simulink model "Control_test"  (R2014b)
settings: Solver=FixedStepDiscrete  StartTime=0.0  StopTime=Inf  FixedStep=0.001  RelTol=1e-3
PostLoadFcn:
  | , if any(exist('dsrtsu_mdlpostloadfcn', 'file') == [2, 3, 6]), try dsrtsu_mdlpostloadfcn('Execute', bdroot); catch fprintf('Error in PostLoadFcn (dsrtsu_mdlpostloadfcn) for model "%s":\n %s\n', bdroot, lasterr); end, end,
undefined symbols (not defined in the file or in its folder): dtLocal, slcm
libraries: rtican x163, simulink x14
(part 8 of 34)

== system Control_test/OutputProcessing/SPAS5 ==
  T_Spas_Stat : Inport
  T_Spas_TM_CTRL_Mode : Inport  Port=2
  T_Spas_TM_Cmd : Inport  Port=3
  T_Spas_AliveCnt : Inport  Port=4
  L_SPAS5 : rtican/RTICAN Transmit (TX)   Reserved1=[]  Reserved2=[]  Reserved3=[]  Reserved4=[]  SfcnMessage=[]  Msg_Struct=[]  BoardTypeNo=[]  BoardNo=[]  ChannelNo=[]  Parameters=[]  DialogFcn=[]  UnitName=[]  Revision=[]  UnitValues=[]  DSProperties=struct('RTI',struct('Version',uint32(5),'BlockType',struct('isSLSource',uint8(1),'isSLSink',uint8(1),'isHWSource',uint8(0),'isHWSink',uint8(0),'isSetup',uint8(0),'isInline',uint8(1),'isNonInline',uint8(0),'isInterrupt',uint8(0),'isChannelwise',uint8(0)),'IOBoardType','RTICAN','UnitType','MESSAGE','Identifier','TX','DialogType','MSVC','BlockSet','RTICAN','SlaveProcessor','CAN'))  RTIBlockInterface=struct('InputPortsWidth',int32([1 1 1 1]),'InputPortsActive',[1 1 1 1],'InputPortsName',{{'T_Spas_Stat','T_Spas_TM_CTRL_Mode','T_Spas_TM_Cmd','T_Spas_AliveCnt'}},'InputPortsDataType',{{'SS_DOUBLE','SS_DOUBLE','SS_DOUBLE','SS_DOUBLE'}},'OutputPortsWidth',int32(0),'OutputPortsActive',0,'OutputPortsName',{{''}},'DialogFcn','rtican_message_interface_gui','BlockDisplay',{{'','center'}},'IconTransparency','on','InitLevel',3,'BlockName',struct('Token',{{'L_SPAS5'}}),'SampleTime',{{0.1}},'TriggerPort',{{'none'}},'EnablePort',{{'none'}})  RTIBlockParameters=struct('BoardTypeNo',{{1,'OFF',[]}},'BoardNo',{{1,'ON',[1 16]}},'ChannelNo',{{1,'ON',[1 2]}},'Parameters',{{struct('DataFileSupport',struct('DataFileSelectedMaster',1,'DataFileSelectedLocal',1,'DataFileName',['c:\users\mpc\dropbox\hyundai car setup\01_dbc_files\hmc_can_for_ucb_v2.dbc|c:\users\mpc\dropbox\hyundai car setup\mobileye spec new\mobileye_mando_camera_ucb_v2.dbc|'],'DataFileDate',{{{['26-Nov-2014 10:54:28']},{['18-Sep-2013 10:55:24']}}},'SelectedFile','c:\users\mpc_car\documents\github\mpc-car\dbcfiles\hmc_can_for_ucb_v2.dbc'),'Options',struct('StatusSelected',0,'TimeSelected',0,'DeltaTimeSelected',0,'DelayTimeSelected',0,'DelayTimeTXCommandSelected',0,'EncodeSetUnusedBitsToOne',0,'EnableMsgLoopback',0,'TriggerPort',struct('Selected',0,'TriggerType',0),'EnablePortSelected',0,'SignalOnPortnameSelected',1,'UserCoding',struct('Selected',0,'InterfaceFile','UserEncodingFile','FcnName','UserEncodeFcn','InportSelected',0,'InportWidth',1,'OutportSelected',0,'OutportWidth',1),'TerminationMsg',struct('Selected',0,'Byte0_7','0'),'InitialMsg',struct('Selected',0,'Byte0_7','0')),'Message',struct('MsgOnBlocknameSelected',1,'MsgName','L_SPAS5','MsgIdFormat',0,'MsgId',1584,'MsgLength',8,'NumSignals',4,'SampleTime',0.1,'StartTime',struct('Selected',0,'Value',0),'AutoRepeatTime',struct('Selected',0,'Value',0.1),'Timeout',struct('Selected',0,'Value',0.1),'DelayTime',struct('Selected',0,'Value',0.1),'Signal',struct('SgnName',{'T_Spas_Stat','T_Spas_TM_CTRL_Mode','T_Spas_TM_Cmd','T_Spas_AliveCnt'},'SgnStartBit',{0,8,16,24},'SgnLength',{4,4,4,8},'SgnType',{0,0,0,0},'ModeValue',{-1,-1,-1,-1},'DataType',{1,1,1,0},'ByteLayout',{0,0,0,0},'Factor',{1,1,1,1},'Offset',{0,0,0,0},'SgnComment',{{''},{''},{''},{''}},'SgnUnit',{'','','',''},'Min',{0,0,0,0},'Max',{0,0,0,0},'SLDataType',{'SS_DOUBLE','SS_DOUBLE','SS_DOUBLE','SS_DOUBLE'}),'MsgIdNumFormat',1,'MsgComment',{{''}}),'Version',1.2,'general',struct('isFromLib',0)),'OFF',[]}},'GroupId',{{struct('Group',{{'RTICAN'}},'No',1,'Behavior',{{'NAMECHANGE'}},'BlockType',{{'SINK'}},'NameChangeFlag',0),'OFF',[]}},'SFcnRTICANMessage',{{struct('MsgType','TX','SFcnPortType','Scalar','MsgName','L_SPAS5','MsgIdFormat','STD','MsgId',1584,'MsgLength',8,'NumSignals',4,'SampleTime',0.1,'StartTime',struct('Selected','no','Value',0),'AutoRepeatTime',struct('Selected','no','Value',0.1),'Timeout',struct('Selected','no','Value',0.1),'Signal',struct('SgnName',{'T_Spas_Stat','T_Spas_TM_CTRL_Mode','T_Spas_TM_Cmd','T_Spas_AliveCnt'},'SgnStartBit',{0,8,16,24},'SgnLength',{4,4,4,8},'SgnType',{'standard','standard','standard','standard'},'ModeValue',{-1,-1,-1,-1},'DataType',{['signed int'],['signed int'],['signed int'],['unsigned int']},'ByteLayout',{['little endian'],['little endian'],['little endian'],['little endian']},'Factor',{1,1,1,1},'Offset',{0,0,0,0},'SLDataType',{'SS_DOUBLE','SS_DOUBLE','SS_DOUBLE','SS_DOUBLE'}),'StatusSelected','no','TimeSelected','no','DeltaTimeSelected','no','DelayTimeSelected','no','DelayTimeTXCommandSelected','no','EncodeSetUnusedBitsToOne','no','EnableMsgLoopback','no','TriggerPort',struct('Selected','no','TriggerType',0),'EnablePortSelected','no','UserCoding',struct('Selected','no','InterfaceFile','UserEncodingFile','FcnName','UserEncodeFcn','InportSelected','no','InportWidth',1,'OutportSelected','no','OutportWidth',1),'TerminationMsg',struct('Selected','no','Byte0','0x00','Byte1','0x00','Byte2','0x00','Byte3','0x00','Byte4','0x00','Byte5','0x00','Byte6','0x00','Byte7','0x00'),'InitialMsg',struct('Selected','no','Byte0','0x00','Byte1','0x00','Byte2','0x00','Byte3','0x00','Byte4','0x00','Byte5','0x00','Byte6','0x00','Byte7','0x00'),'BoardType','DS1','BoardNo',1,'ControllerNo',1),'OFF',[]}},'TLCFileName',{{'rtican_tx_message','OFF',[]}})  RTISFcnParameters=struct('SFcnRTICANMessage','struct','TLCFileName','char')  RTIBlockParaDefault=struct('BoardTypeNo',4302,'BoardNo',1,'ChannelNo',1,'Parameters',struct('DataFileSupport',struct('DataFileSelectedMaster',0,'DataFileSelectedLocal',0,'DataFileName','','DataFileDate','','SelectedFile',['<no file selected>']),'Options',struct('StatusSelected',1,'TimeSelected',1,'DeltaTimeSelected',1,'DelayTimeSelected',1,'DelayTimeTXCommandSelected',0,'EncodeSetUnusedBitsToOne',0,'EnableMsgLoopback',0,'TriggerPort',struct('Selected',0,'TriggerType','rising'),'EnablePortSelected',0,'SignalOnPortnameSelected',1,'UserCoding',struct('Selected',0,'InterfaceFile','UserEncodingFile','FcnName','UserEncodeFcn','InportSelected',0,'InportWidth',1,'OutportSelected',0,'OutportWidth',1),'TerminationMsg',struct('Selected',0,'Byte0_7','0'),'InitialMsg',struct('Selected',0,'Byte0_7','0')),'Message',struct('MsgOnBlocknameSelected',0,'MsgName',['TX Message'],'MsgIdFormat',0,'MsgId',100,'MsgLength',8,'NumSignals',1,'SampleTime',-1,'StartTime',struct('Selected',0,'Value',0),'AutoRepeatTime',struct('Selected',0,'Value',0.1),'Timeout',struct('Selected',0,'Value',0.1),'DelayTime',struct('Selected',0,'Value',0.1),'Signal',struct('SgnName',['TX signal'],'SgnStartBit',0,'SgnLength',8,'SgnType',0,'ModeValue',-1,'DataType',0,'SLDataType','SS_DOUBLE','ByteLayout',0,'Factor',1,'Offset',0,'Min',0,'Max',255,'SgnComment',{{}},'SgnUnit',''),'MsgIdNumFormat',0,'MsgComment',{{''}}),'Version',1.2,'general',struct('isFromLib',1)),'GroupId',struct('Group',{{'RTICAN'}},'No',1,'Behavior',{{'NAMECHANGE'}},'BlockType',{{'SINK'}},'NameChangeFlag',0),'SFcnRTICANMessage',struct('MsgType','TX','MsgName',['TX Message'],'MsgIdFormat','STD','MsgId',100,'MsgLength',2,'NumSignals',1,'SampleTime',-1,'StartTime',struct('Selected','no','Value',0),'AutoRepeatTime',struct('Selected','no','Value',0.1),'Timeout',struct('Selected','no','Value',0.1),'DelayTime',struct('Selected','no','Value',0.1),'Signal',struct('SgnName',['TX signal'],'SgnStartBit',0,'SgnLength',8,'SgnType','standard','ModeValue',-1,'DataType',['unsigned int'],'ByteLayout',['little endian'],'SLDataType','SS_DOUBLE','Factor',1,'Offset',0),'StatusSelected','yes','TimeSelected','yes','DeltaTimeSelected','yes','DelayTimeSelected','yes','EnablePortSelected','no','EnableMsgLoopback','no','DelayTimeTXCommandSelected','no','EncodeSetUnusedBitsToOne','no','UserCoding',struct('Selected','no','InterfaceFile','UserDecodingFile','FcnName','UserDecodeFcn','InportSelected','no','InportWidth',1,'OutportSelected','no','OutportWidth',1),'TerminationMsg',struct('Selected','no','Byte0','0x00','Byte1','0x00','Byte2','0x00','Byte3','0x00','Byte4','0x00','Byte5','0x00','Byte6','0x00','Byte7','0x00'),'InitialMsg',struct('Selected','no','Byte0','0x00','Byte1','0x00','Byte2','0x00','Byte3','0x00','Byte4','0x00','Byte5','0x00','Byte6','0x00','Byte7','0x00'),'TriggerPort',struct('Selected','no','TriggerType','rising'),'BoardType','DS4302','BoardNo',1,'ControllerNo',1,'SFcnPortType','Scalar'),'TLCFileName','rtican_tx_message')
      settings: AttributesFormatString=Group Id: RTICAN1\n
  Rate Transition{1..4} (4 alike) : RateTransition  OutPortSampleTime=0.1
  wires:
  T_Spas_Stat/1 -> Rate Transition4/1
  T_Spas_TM_CTRL_Mode/1 -> Rate Transition3/1
  T_Spas_TM_Cmd/1 -> Rate Transition1/1
  Rate Transition1/1 -> L_SPAS5/3
  Rate Transition3/1 -> L_SPAS5/2
  Rate Transition4/1 -> L_SPAS5/1
  Rate Transition2/1 -> L_SPAS5/4
  T_Spas_AliveCnt/1 -> Rate Transition2/1

== system Control_test/OutputProcessing/TM_AliveCnt ==
  Trigger : TriggerPort  PortDimensions=1
  Add : Sum
  Constant : Constant
  Constant1 : Constant  Value=0
  Switch1 : Switch  Criteria=u2 > Threshold  Threshold=255
  Unit Delay : UnitDelay  SampleTime=-1
  T_Spas_AliveCnt : Outport
  wires:
  Constant/1 -> Add/1
  Constant1/1 -> Switch1/1
  Add/1 -> Switch1/2, Switch1/3
  Switch1/1 -> Unit Delay/1, T_Spas_AliveCnt/1
  Unit Delay/1 -> Add/2

== system Control_test/OutputProcessing/VehicleCanProcessing ==
  In1 : Inport
  delta_f [rad] : Inport  Port=2
  DriverOverride_flag : Inport  Port=3
  torque [Nm] : Inport  Port=4
  " " : Gain
  " 1" : Gain
  Active Flag : Constant  Value=0
  Add : Sum
  Add1 : Sum
  Bus Selector : BusSelector  OutputSignals=Vehicle Data.EMS1.ipEmsVehSpd[kph],Vehicle Data.SAS1Data.ipStrAng[deg]
  GearRatio : Gain  Gain=14.5
  LKAS2 : Subsystem
  Req Steering Angle [deg] : Constant  Value=0
  Saturation : Saturate  UpperLimit=360  LowerLimit=-360
  Switch1 : Switch  Threshold=0.5
  default1 : Constant  Value=0
  rad2deg : Gain  Gain=(180/pi)
  steerOffDeg : Constant  Value=0
  tag scope: SteerActiveFlag=global
  wires:
  In1/1 -> Bus Selector/1
  Bus Selector/1 -> LKAS2/3(Vs)  "<ipEmsVehSpd[kph]>"
  Bus Selector/2 -> LKAS2/4(SteeringAngle)  "<ipStrAng[deg]>"
  Req Steering Angle [deg]/1 -> " 1"/1
  Add/1 -> LKAS2/1(Req Steering Angle[deg])
  " "/1 -> LKAS2/2(Active_Flag)  "in_enable"
  " 1"/1 -> Add/2  "Req_Steering_Angle_deg"
  Add1/1 -> Add/1
  delta_f [rad]/1 -> rad2deg/1
  rad2deg/1 -> GearRatio/1
  Switch1/1 -> " "/1
  default1/1 -> Switch1/1
  DriverOverride_flag/1 -> Switch1/2
  Active Flag/1 -> Switch1/3, [SteerActiveFlag]
  GearRatio/1 -> Saturation/1
  Saturation/1 -> Add1/1  "commanded_steering"
  steerOffDeg/1 -> Add1/2
  torque [Nm]/1 -> LKAS2/5(Req Steering Tq [Nm])

== system Control_test/RTI Data/RTI Data Store ==
  RTI Data Store : Subsystem  mask(RTI_DATA_STORE){}
      mask help:
      | RTI Data Store Block. This block is used by RTI to store internal model dependent data. Deleting this block will result in data loss.
      |
      | NEVER DELETE, COPY, OR MODIFY THIS BLOCK!
      mask Help:
      | RTI Data Store Block. This block is used by RTI to store internal model dependent data. Deleting this block will result in data loss.
      | 
      | NEVER DELETE, COPY, OR MODIFY THIS BLOCK!
      mask Display: text(0.5, 0.5, ' ', 'HorizontalAlignment', 'center');

== system Control_test/SensorFusion/Map-based Localization ==
  In1 : Inport
  Add : Sum
  Bus Selector1 : BusSelector  OutputSignals=IMU_data.signal2.PosLon,IMU_data.signal2.PosLat,IMU_data.signal1.AngleHeading,Vehicle Data.WhlSpdData.ipVehSpdWhl[m/s]
  INS Reference Change : MATLAB Function
      settings: RTWSystemCode=Inline
  Mux1 : Mux  Inputs=3
  Mux4 : Mux  Inputs=2
  OffsetX : Constant  Value=0
  OffsetY : Constant  Value=0
  gain1 : Gain
  gain2 : Gain
  OutMap : Outport
  wires:
  Add/1 -> Mux1/1
  OffsetY/1 -> gain2/1
  OffsetX/1 -> gain1/1
  Mux4/1 -> Add/1
  gain1/1 -> Mux4/1  "MapOffsetX"
  gain2/1 -> Mux4/2  "MapOffsetY"
  In1/1 -> Bus Selector1/1
  INS Reference Change/1(GPS_Local_Pos) -> Add/2
  INS Reference Change/2(INS_Heading) -> Mux1/2
  Bus Selector1/4 -> Mux1/3  "<ipVehSpdWhl[m/s]>"
  Bus Selector1/1 -> INS Reference Change/1(PosLon)  "<PosLon>"
  Bus Selector1/2 -> INS Reference Change/2(PosLat)  "<PosLat>"
  Bus Selector1/3 -> INS Reference Change/3(AngleHeading)  "<AngleHeading>"
  Mux1/1 -> OutMap/1

== system Control_test/InputProcessing/CameraCanProcessing/ME_Lane_Additional_Data_1 ==
  Bus Creator : BusCreator  Inputs=14
  ME_Lane_Additional_Data_1 : rtican/RTICAN Receive (RX)   Reserved1=[]  Reserved2=[]  Reserved3=[]  Reserved4=[]  SfcnMessage=[]  Msg_Struct=[]  BoardTypeNo=[]  BoardNo=[]  ChannelNo=[]  Parameters=[]  DialogFcn=[]  UnitName=[]  Revision=[]  UnitValues=[]  DSProperties=struct('RTI',struct('Version',uint32(5),'BlockType',struct('isSLSource',uint8(1),'isSLSink',uint8(1),'isHWSource',uint8(0),'isHWSink',uint8(0),'isSetup',uint8(0),'isInline',uint8(1),'isNonInline',uint8(0),'isInterrupt',uint8(0),'isChannelwise',uint8(0)),'IOBoardType','RTICAN','UnitType','MESSAGE','Identifier','RX','DialogType','MSVC','BlockSet','RTICAN','SlaveProcessor','CAN'))  RTIBlockInterface=struct('OutputPortsWidth',int32([1 1 1 1 1 1 1 1 1 1 1 1 1 1]),'OutputPortsActive',[1 1 1 1 1 1 1 1 1 1 1 1 1 1],'OutputPortsName',{{'Rh_Neightbor_Avail','Lh_Neightbor_Avail','Rh_Neightbor_Type','Lh_Neightbor_Type','Alive_Counter_MELaneAddData','Rh_Guardrail','Lh_Guardrail','RightLanePrediction','LeftLanePrediction','HighwayExit','RightLaneColorInfo','LeftLaneColorInfo','Lh_ViewRange_StartPoint','Rh_ViewRange_StartPoint'}},'OutputPortsDataType',{{'SS_DOUBLE','SS_DOUBLE','SS_DOUBLE','SS_DOUBLE','SS_DOUBLE','SS_DOUBLE','SS_DOUBLE','SS_DOUBLE','SS_DOUBLE','SS_DOUBLE','SS_DOUBLE','SS_DOUBLE','SS_DOUBLE','SS_DOUBLE'}},'OutputPortsLabel',{{'Rh_Neightbor_Avail','Lh_Neightbor_Avail','Rh_Neightbor_Type','Lh_Neightbor_Type','Alive_Counter_MELaneAddData','Rh_Guardrail','Lh_Guardrail','RightLanePrediction','LeftLanePrediction','HighwayExit','RightLaneColorInfo','LeftLaneColorInfo','Lh_ViewRange_StartPoint','Rh_ViewRange_StartPoint'}},'OutputPortsLabelMode','ON','InputPortsWidth',int32(0),'InputPortsActive',0,'DialogFcn','rtican_message_interface_gui','BlockDisplay',{{'','center'}},'IconTransparency','on','ParameterTunableNames',{{}},'InitLevel',3,'BlockName',struct('Token',{{'ME_Lane_Additional_Data_1'}}),'SampleTime',{{0.01}},'TriggerPort',{{'none'}},'EnablePort',{{'none'}})  RTIBlockParameters=struct('BoardTypeNo',{{1,'OFF',[]}},'BoardNo',{{1,'ON',[1 16]}},'ChannelNo',{{2,'ON',[1 2]}},'Parameters',{{struct('DataFileSupport',struct('DataFileSelectedMaster',1,'DataFileSelectedLocal',1,'DataFileName',['c:\users\mpc\desktop\hyundai car setup\rt2000_can_mod.dbc|c:\users\mpc\desktop\hyundai car setup\mobileye spec new\mobileye_mando_camera_ucb_v2.dbc|'],'DataFileDate',['18-Sep-2013 17:55:24'],'SelectedFile','..\..\dbcfiles\mobileye_mando_camera_ucb_v2.dbc','InterfaceFcn','rtican_dbc_file_parser'),'Options',struct('StatusSelected',0,'TimeSelected',0,'DeltaTimeSelected',0,'BytePortSelected',0,'MessageLengthSelected',0,'TriggerPort',struct('Selected',0,'TriggerType',0),'UserCoding',struct('Selected',0,'InterfaceFile','UserDecodingFile','FcnName','UserDecodeFcn','InportSelected',0,'InportWidth',1,'OutportSelected',0,'OutportWidth',1),'EnablePortSelected',0,'SignalOnPortnameSelected',1,'UseRXService',0),'Message',struct('MsgOnBlocknameSelected',1,'MsgName','ME_Lane_Additional_Data_1','MsgIdFormat',0,'MsgId',1901,'MsgLength',8,'NumSignals',14,'SampleTime',0.01,'Signal',struct('SgnName',{'Rh_Neightbor_Avail','Lh_Neightbor_Avail','Rh_Neightbor_Type','Lh_Neightbor_Type','Alive_Counter_MELaneAddData','Rh_Guardrail','Lh_Guardrail','RightLanePrediction','LeftLanePrediction','HighwayExit','RightLaneColorInfo','LeftLaneColorInfo','Lh_ViewRange_StartPoint','Rh_ViewRange_StartPoint'},'SgnStartBit',{0,4,8,12,16,18,19,24,25,26,28,30,32,48},'SgnLength',{4,4,4,4,2,1,1,1,1,1,2,2,16,16},'ByteLayout',{0,0,0,0,0,0,0,0,0,0,0,0,0,0},'Factor',{1,1,1,1,1,1,1,1,1,1,1,1,0.01,0.01},'Offset',{0,0,0,0,0,0,0,0,0,0,0,0,0,0},'SgnComment',{'','','','','','','','','','','','','',''},'SgnUnit',{'','','','','','','','','','','','','',''},'Min',{0,0,0,0,0,0,0,0,0,0,0,0,0,0},'Max',{0,0,0,0,0,0,0,0,0,0,0,0,0,0},'SgnType',{0,0,0,0,0,0,0,0,0,0,0,0,0,0},'SLDataType',{'SS_DOUBLE','SS_DOUBLE','SS_DOUBLE','SS_DOUBLE','SS_DOUBLE','SS_DOUBLE','SS_DOUBLE','SS_DOUBLE','SS_DOUBLE','SS_DOUBLE','SS_DOUBLE','SS_DOUBLE','SS_DOUBLE','SS_DOUBLE'},'DataType',{0,0,0,0,0,0,0,0,0,0,0,0,0,0},'ModeValue',{-1,-1,-1,-1,-1,-1,-1,-1,-1,-1,-1,-1,-1,-1}),'MsgIdNumFormat',0,'MsgComment',{{''}}),'Version',1.2,'general',struct('isFromLib',0)),'OFF',[]}},'GroupId',{{struct('Group',{{'RTICAN'}},'No',2,'Behavior',{{'NAMECHANGE'}},'BlockType',{{'SINK'}},'NameChangeFlag',0),'OFF',[]}},'SFcnRTICANMessage',{{struct('MsgType','RX','SFcnPortType','Scalar','MsgName','ME_Lane_Additional_Data_1','MsgIdFormat','STD','MsgId',1901,'MsgLength',8,'NumSignals',14,'SampleTime',0.01,'Signal',struct('SgnName',{'Rh_Neightbor_Avail','Lh_Neightbor_Avail','Rh_Neightbor_Type','Lh_Neightbor_Type','Alive_Counter_MELaneAddData','Rh_Guardrail','Lh_Guardrail','RightLanePrediction','LeftLanePrediction','HighwayExit','RightLaneColorInfo','LeftLaneColorInfo','Lh_ViewRange_StartPoint','Rh_ViewRange_StartPoint'},'SgnStartBit',{0,4,8,12,16,18,19,24,25,26,28,30,32,48},'SgnLength',{4,4,4,4,2,1,1,1,1,1,2,2,16,16},'ByteLayout',{['little endian'],['little endian'],['little endian'],['little endian'],['little endian'],['little endian'],['little endian'],['little endian'],['little endian'],['little endian'],['little endian'],['little endian'],['little endian'],['little endian']},'Factor',{1,1,1,1,1,1,1,1,1,1,1,1,0.01,0.01},'Offset',{0,0,0,0,0,0,0,0,0,0,0,0,0,0},'SgnType',{'standard','standard','standard','standard','standard','standard','standard','standard','standard','standard','standard','standard','standard','standard'},'SLDataType',{'SS_DOUBLE','SS_DOUBLE','SS_DOUBLE','SS_DOUBLE','SS_DOUBLE','SS_DOUBLE','SS_DOUBLE','SS_DOUBLE','SS_DOUBLE','SS_DOUBLE','SS_DOUBLE','SS_DOUBLE','SS_DOUBLE','SS_DOUBLE'},'DataType',{['unsigned int'],['unsigned int'],['unsigned int'],['unsigned int'],['unsigned int'],['unsigned int'],['unsigned int'],['unsigned int'],['unsigned int'],['unsigned int'],['unsigned int'],['unsigned int'],['unsigned int'],['unsigned int']},'ModeValue',{-1,-1,-1,-1,-1,-1,-1,-1,-1,-1,-1,-1,-1,-1}),'StatusSelected','no','TimeSelected','no','DeltaTimeSelected','no','BytePortSelected','no','MessageLengthSelected','no','TriggerPort',struct('Selected','no','TriggerType',0),'UserCoding',struct('Selected','no','InterfaceFile','UserDecodingFile','FcnName','UserDecodeFcn','InportSelected','no','InportWidth',1,'OutportSelected','no','OutportWidth',1),'EnablePortSelected','no','UseRXService','no','BoardType','DS1','BoardNo',1,'ControllerNo',2),'OFF',[]}},'TLCFileName',{{'rtican_rx_message','OFF',[]}})  RTISFcnParameters=struct('SFcnRTICANMessage','struct','TLCFileName','char')  RTIBlockParaDefault=struct('BoardTypeNo',4302,'BoardNo',1,'ChannelNo',1,'Parameters',struct('DataFileSupport',struct('DataFileSelectedMaster',0,'DataFileSelectedLocal',0,'DataFileName','','DataFileDate','','SelectedFile',['<no file selected>']),'Options',struct('StatusSelected',1,'TimeSelected',1,'DeltaTimeSelected',1,'BytePortSelected',0,'MessageLengthSelected',0,'TriggerPort',struct('Selected',0,'TriggerType','rising'),'UserCoding',struct('Selected',0,'InterfaceFile','UserDecodingFile','FcnName','UserDecodeFcn','InportSelected',0,'InportWidth',1,'OutportSelected',0,'OutportWidth',1),'EnablePortSelected',0,'SignalOnPortnameSelected',1,'UseRXService',0),'Message',struct('MsgOnBlocknameSelected',0,'MsgName',['RX Message'],'MsgIdFormat',0,'MsgId',100,'MsgLength',8,'NumSignals',1,'SampleTime',-1,'Signal',struct('SgnName',['RX signal'],'SgnStartBit',0,'SgnLength',8,'SgnType',0,'ModeValue',-1,'DataType',0,'SLDataType','SS_DOUBLE','ByteLayout',0,'Factor',1,'Offset',0,'Min',0,'Max',255,'SgnComment',{{}},'SgnUnit',''),'MsgIdNumFormat',0,'MsgComment',{{''}}),'Version',1.2,'general',struct('isFromLib',1)),'GroupId',struct('Group',{{'RTICAN'}},'No',1,'Behavior',{{'NAMECHANGE'}},'BlockType',{{'SINK'}},'NameChangeFlag',0),'SFcnRTICANMessage',struct('MsgType','RX','MsgName',['RX Message'],'MsgIdFormat','STD','MsgId',100,'MsgLength',8,'NumSignals',1,'SampleTime',-1,'Signal',struct('SgnName',['RX signal'],'SgnStartBit',0,'SgnLength',8,'SgnType','standard','ModeValue',-1,'DataType',['unsigned int'],'ByteLayout',['little endian'],'SLDataType','SS_DOUBLE','Factor',1,'Offset',0),'StatusSelected','yes','TimeSelected','yes','DeltaTimeSelected','yes','BytePortSelected','no','MessageLengthSelected','no','EnablePortSelected','no','UserCoding',struct('Selected','no','InterfaceFile','UserDecodingFile','FcnName','UserDecodeFcn','InportSelected','no','InportWidth',1,'OutportSelected','no','OutportWidth',1),'TriggerPort',struct('Selected','no','TriggerType','rising'),'UseRXService','no','BoardType','DS4302','BoardNo',1,'ControllerNo',1,'SFcnPortType','Scalar'),'TLCFileName','rtican_rx_message')
      settings: AttributesFormatString=Group Id: RTICAN2\n
  ME_Lane_Additional_Data_1_CAN : Outport
  wires:
  Bus Creator/1 -> ME_Lane_Additional_Data_1_CAN/1
  ME_Lane_Additional_Data_1/1 -> Bus Creator/1  "Rh_Neightbor_Avail"
  ME_Lane_Additional_Data_1/2 -> Bus Creator/2  "Lh_Neightbor_Avail"
  ME_Lane_Additional_Data_1/3 -> Bus Creator/3  "Rh_Neightbor_Type"
  ME_Lane_Additional_Data_1/4 -> Bus Creator/4  "Lh_Neightbor_Type"
  ME_Lane_Additional_Data_1/5 -> Bus Creator/5  "Alive_Counter_MELaneAddData"
  ME_Lane_Additional_Data_1/6 -> Bus Creator/6  "Rh_Guardrail"
  ME_Lane_Additional_Data_1/7 -> Bus Creator/7  "Lh_Guardrail"
  ME_Lane_Additional_Data_1/8 -> Bus Creator/8  "RightLanePrediction"
  ME_Lane_Additional_Data_1/9 -> Bus Creator/9  "LeftLanePrediction"
  ME_Lane_Additional_Data_1/10 -> Bus Creator/10  "HighwayExit"
  ME_Lane_Additional_Data_1/11 -> Bus Creator/11  "RightLaneColorInfo"
  ME_Lane_Additional_Data_1/12 -> Bus Creator/12  "LeftLaneColorInfo"
  ME_Lane_Additional_Data_1/13 -> Bus Creator/13  "Lh_ViewRange_StartPoint"
  ME_Lane_Additional_Data_1/14 -> Bus Creator/14  "Rh_ViewRange_StartPoint"

== system Control_test/InputProcessing/CameraCanProcessing/ME_Lane_Additional_Data_2 ==
  Bus Creator : BusCreator  Inputs=5
  ME_Lane_Additional_Data_2 : rtican/RTICAN Receive (RX)   Reserved1=[]  Reserved2=[]  Reserved3=[]  Reserved4=[]  SfcnMessage=[]  Msg_Struct=[]  BoardTypeNo=[]  BoardNo=[]  ChannelNo=[]  Parameters=[]  DialogFcn=[]  UnitName=[]  Revision=[]  UnitValues=[]  DSProperties=struct('RTI',struct('Version',uint32(5),'BlockType',struct('isSLSource',uint8(1),'isSLSink',uint8(1),'isHWSource',uint8(0),'isHWSink',uint8(0),'isSetup',uint8(0),'isInline',uint8(1),'isNonInline',uint8(0),'isInterrupt',uint8(0),'isChannelwise',uint8(0)),'IOBoardType','RTICAN','UnitType','MESSAGE','Identifier','RX','DialogType','MSVC','BlockSet','RTICAN','SlaveProcessor','CAN'))  RTIBlockInterface=struct('OutputPortsWidth',int32([1 1 1 1 1]),'OutputPortsActive',[1 1 1 1 1],'OutputPortsName',{{'Alive_Counter_MELaneAddData','Lh_Neighbor_Pos','Lh_Neighbor_Model_B','Lh_Neighbor_Model_A','Lh_Neighbor_Model_dA'}},'OutputPortsDataType',{{'SS_DOUBLE','SS_DOUBLE','SS_DOUBLE','SS_DOUBLE','SS_DOUBLE'}},'OutputPortsLabel',{{'Alive_Counter_MELaneAddData','Lh_Neighbor_Pos','Lh_Neighbor_Model_B','Lh_Neighbor_Model_A','Lh_Neighbor_Model_dA'}},'OutputPortsLabelMode','ON','InputPortsWidth',int32(0),'InputPortsActive',0,'DialogFcn','rtican_message_interface_gui','BlockDisplay',{{'','center'}},'IconTransparency','on','ParameterTunableNames',{{}},'InitLevel',3,'BlockName',struct('Token',{{'ME_Lane_Additional_Data_2'}}),'SampleTime',{{0.01}},'TriggerPort',{{'none'}},'EnablePort',{{'none'}})  RTIBlockParameters=struct('BoardTypeNo',{{1,'OFF',[]}},'BoardNo',{{1,'ON',[1 16]}},'ChannelNo',{{2,'ON',[1 2]}},'Parameters',{{struct('DataFileSupport',struct('DataFileSelectedMaster',1,'DataFileSelectedLocal',1,'DataFileName',['c:\users\mpc\desktop\hyundai car setup\rt2000_can_mod.dbc|c:\users\mpc\desktop\hyundai car setup\mobileye spec new\mobileye_mando_camera_ucb_v2.dbc|'],'DataFileDate',['18-Sep-2013 17:55:24'],'SelectedFile','..\..\dbcfiles\mobileye_mando_camera_ucb_v2.dbc','InterfaceFcn','rtican_dbc_file_parser'),'Options',struct('StatusSelected',0,'TimeSelected',0,'DeltaTimeSelected',0,'BytePortSelected',0,'MessageLengthSelected',0,'TriggerPort',struct('Selected',0,'TriggerType',0),'UserCoding',struct('Selected',0,'InterfaceFile','UserDecodingFile','FcnName','UserDecodeFcn','InportSelected',0,'InportWidth',1,'OutportSelected',0,'OutportWidth',1),'EnablePortSelected',0,'SignalOnPortnameSelected',1,'UseRXService',0),'Message',struct('MsgOnBlocknameSelected',1,'MsgName','ME_Lane_Additional_Data_2','MsgIdFormat',0,'MsgId',1902,'MsgLength',8,'NumSignals',5,'SampleTime',0.01,'Signal',struct('SgnName',{'Alive_Counter_MELaneAddData','Lh_Neighbor_Pos','Lh_Neighbor_Model_B','Lh_Neighbor_Model_A','Lh_Neighbor_Model_dA'},'SgnStartBit',{0,8,16,32,48},'SgnLength',{2,8,16,16,16},'ByteLayout',{0,0,0,0,0},'Factor',{1,0.05,1,1,1},'Offset',{0,0,0,0,0},'SgnComment',{'','','','',''},'SgnUnit',{'','','','',''},'Min',{0,0,0,0,0},'Max',{0,0,0,0,0},'SgnType',{0,0,0,0,0},'SLDataType',{'SS_DOUBLE','SS_DOUBLE','SS_DOUBLE','SS_DOUBLE','SS_DOUBLE'},'DataType',{0,0,1,1,1},'ModeValue',{-1,-1,-1,-1,-1}),'MsgIdNumFormat',0,'MsgComment',{{''}}),'Version',1.2,'general',struct('isFromLib',0)),'OFF',[]}},'GroupId',{{struct('Group',{{'RTICAN'}},'No',2,'Behavior',{{'NAMECHANGE'}},'BlockType',{{'SINK'}},'NameChangeFlag',0),'OFF',[]}},'SFcnRTICANMessage',{{struct('MsgType','RX','SFcnPortType','Scalar','MsgName','ME_Lane_Additional_Data_2','MsgIdFormat','STD','MsgId',1902,'MsgLength',8,'NumSignals',5,'SampleTime',0.01,'Signal',struct('SgnName',{'Alive_Counter_MELaneAddData','Lh_Neighbor_Pos','Lh_Neighbor_Model_B','Lh_Neighbor_Model_A','Lh_Neighbor_Model_dA'},'SgnStartBit',{0,8,16,32,48},'SgnLength',{2,8,16,16,16},'ByteLayout',{['little endian'],['little endian'],['little endian'],['little endian'],['little endian']},'Factor',{1,0.05,1,1,1},'Offset',{0,0,0,0,0},'SgnType',{'standard','standard','standard','standard','standard'},'SLDataType',{'SS_DOUBLE','SS_DOUBLE','SS_DOUBLE','SS_DOUBLE','SS_DOUBLE'},'DataType',{['unsigned int'],['unsigned int'],['signed int'],['signed int'],['signed int']},'ModeValue',{-1,-1,-1,-1,-1}),'StatusSelected','no','TimeSelected','no','DeltaTimeSelected','no','BytePortSelected','no','MessageLengthSelected','no','TriggerPort',struct('Selected','no','TriggerType',0),'UserCoding',struct('Selected','no','InterfaceFile','UserDecodingFile','FcnName','UserDecodeFcn','InportSelected','no','InportWidth',1,'OutportSelected','no','OutportWidth',1),'EnablePortSelected','no','UseRXService','no','BoardType','DS1','BoardNo',1,'ControllerNo',2),'OFF',[]}},'TLCFileName',{{'rtican_rx_message','OFF',[]}})  RTISFcnParameters=struct('SFcnRTICANMessage','struct','TLCFileName','char')  RTIBlockParaDefault=struct('BoardTypeNo',4302,'BoardNo',1,'ChannelNo',1,'Parameters',struct('DataFileSupport',struct('DataFileSelectedMaster',0,'DataFileSelectedLocal',0,'DataFileName','','DataFileDate','','SelectedFile',['<no file selected>']),'Options',struct('StatusSelected',1,'TimeSelected',1,'DeltaTimeSelected',1,'BytePortSelected',0,'MessageLengthSelected',0,'TriggerPort',struct('Selected',0,'TriggerType','rising'),'UserCoding',struct('Selected',0,'InterfaceFile','UserDecodingFile','FcnName','UserDecodeFcn','InportSelected',0,'InportWidth',1,'OutportSelected',0,'OutportWidth',1),'EnablePortSelected',0,'SignalOnPortnameSelected',1,'UseRXService',0),'Message',struct('MsgOnBlocknameSelected',0,'MsgName',['RX Message'],'MsgIdFormat',0,'MsgId',100,'MsgLength',8,'NumSignals',1,'SampleTime',-1,'Signal',struct('SgnName',['RX signal'],'SgnStartBit',0,'SgnLength',8,'SgnType',0,'ModeValue',-1,'DataType',0,'SLDataType','SS_DOUBLE','ByteLayout',0,'Factor',1,'Offset',0,'Min',0,'Max',255,'SgnComment',{{}},'SgnUnit',''),'MsgIdNumFormat',0,'MsgComment',{{''}}),'Version',1.2,'general',struct('isFromLib',1)),'GroupId',struct('Group',{{'RTICAN'}},'No',1,'Behavior',{{'NAMECHANGE'}},'BlockType',{{'SINK'}},'NameChangeFlag',0),'SFcnRTICANMessage',struct('MsgType','RX','MsgName',['RX Message'],'MsgIdFormat','STD','MsgId',100,'MsgLength',8,'NumSignals',1,'SampleTime',-1,'Signal',struct('SgnName',['RX signal'],'SgnStartBit',0,'SgnLength',8,'SgnType','standard','ModeValue',-1,'DataType',['unsigned int'],'ByteLayout',['little endian'],'SLDataType','SS_DOUBLE','Factor',1,'Offset',0),'StatusSelected','yes','TimeSelected','yes','DeltaTimeSelected','yes','BytePortSelected','no','MessageLengthSelected','no','EnablePortSelected','no','UserCoding',struct('Selected','no','InterfaceFile','UserDecodingFile','FcnName','UserDecodeFcn','InportSelected','no','InportWidth',1,'OutportSelected','no','OutportWidth',1),'TriggerPort',struct('Selected','no','TriggerType','rising'),'UseRXService','no','BoardType','DS4302','BoardNo',1,'ControllerNo',1,'SFcnPortType','Scalar'),'TLCFileName','rtican_rx_message')
      settings: AttributesFormatString=Group Id: RTICAN2\n
  ME_Lane_Additional_Data_2_CAN : Outport
  wires:
  Bus Creator/1 -> ME_Lane_Additional_Data_2_CAN/1
  ME_Lane_Additional_Data_2/1 -> Bus Creator/1  "Alive_Counter_MELaneAddData"
  ME_Lane_Additional_Data_2/2 -> Bus Creator/2  "Lh_Neighbor_Pos"
  ME_Lane_Additional_Data_2/3 -> Bus Creator/3  "Lh_Neighbor_Model_B"
  ME_Lane_Additional_Data_2/4 -> Bus Creator/4  "Lh_Neighbor_Model_A"
  ME_Lane_Additional_Data_2/5 -> Bus Creator/5  "Lh_Neighbor_Model_dA"

== system Control_test/InputProcessing/CameraCanProcessing/ME_Lane_Additional_Data_3 ==
  Bus Creator : BusCreator  Inputs=5
  ME_Lane_Additional_Data_3 : rtican/RTICAN Receive (RX)   Reserved1=[]  Reserved2=[]  Reserved3=[]  Reserved4=[]  SfcnMessage=[]  Msg_Struct=[]  BoardTypeNo=[]  BoardNo=[]  ChannelNo=[]  Parameters=[]  DialogFcn=[]  UnitName=[]  Revision=[]  UnitValues=[]  DSProperties=struct('RTI',struct('Version',uint32(5),'BlockType',struct('isSLSource',uint8(1),'isSLSink',uint8(1),'isHWSource',uint8(0),'isHWSink',uint8(0),'isSetup',uint8(0),'isInline',uint8(1),'isNonInline',uint8(0),'isInterrupt',uint8(0),'isChannelwise',uint8(0)),'IOBoardType','RTICAN','UnitType','MESSAGE','Identifier','RX','DialogType','MSVC','BlockSet','RTICAN','SlaveProcessor','CAN'))  RTIBlockInterface=struct('OutputPortsWidth',int32([1 1 1 1 1]),'OutputPortsActive',[1 1 1 1 1],'OutputPortsName',{{'Alive_Counter_MELaneAddData','Rh_Neighbor_Pos','Rh_Neighbor_Model_B','Rh_Neighbor_Model_A','Rh_Neighbor_Model_dA'}},'OutputPortsDataType',{{'SS_DOUBLE','SS_DOUBLE','SS_DOUBLE','SS_DOUBLE','SS_DOUBLE'}},'OutputPortsLabel',{{'Alive_Counter_MELaneAddData','Rh_Neighbor_Pos','Rh_Neighbor_Model_B','Rh_Neighbor_Model_A','Rh_Neighbor_Model_dA'}},'OutputPortsLabelMode','ON','InputPortsWidth',int32(0),'InputPortsActive',0,'DialogFcn','rtican_message_interface_gui','BlockDisplay',{{'','center'}},'IconTransparency','on','ParameterTunableNames',{{}},'InitLevel',3,'BlockName',struct('Token',{{'ME_Lane_Additional_Data_3'}}),'SampleTime',{{0.01}},'TriggerPort',{{'none'}},'EnablePort',{{'none'}})  RTIBlockParameters=struct('BoardTypeNo',{{1,'OFF',[]}},'BoardNo',{{1,'ON',[1 16]}},'ChannelNo',{{2,'ON',[1 2]}},'Parameters',{{struct('DataFileSupport',struct('DataFileSelectedMaster',1,'DataFileSelectedLocal',0,'DataFileName',['c:\users\mpc\dropbox\hyundai car setup\dbc files\rt2002_can.dbc|c:\users\mpc\dropbox\cpg_test_2014\t4_rfs_demo\hyundai car setup\mobileye spec new\mobileye_mando_camera_ucb_v2.dbc|'],'DataFileDate',{{{['13-Nov-2012 16:29:35']},{['18-Sep-2013 10:55:24']}}},'SelectedFile',['<no file selected>'],'InterfaceFcn','rtican_dbc_file_parser'),'Options',struct('StatusSelected',0,'TimeSelected',0,'DeltaTimeSelected',0,'BytePortSelected',0,'MessageLengthSelected',0,'TriggerPort',struct('Selected',0,'TriggerType',0),'UserCoding',struct('Selected',0,'InterfaceFile','UserDecodingFile','FcnName','UserDecodeFcn','InportSelected',0,'InportWidth',1,'OutportSelected',0,'OutportWidth',1),'EnablePortSelected',0,'SignalOnPortnameSelected',1,'UseRXService',0),'Message',struct('MsgOnBlocknameSelected',1,'MsgName','ME_Lane_Additional_Data_3','MsgIdFormat',0,'MsgId',1903,'MsgLength',8,'NumSignals',5,'SampleTime',0.01,'Signal',struct('SgnName',{'Alive_Counter_MELaneAddData','Rh_Neighbor_Pos','Rh_Neighbor_Model_B','Rh_Neighbor_Model_A','Rh_Neighbor_Model_dA'},'SgnStartBit',{0,8,16,32,48},'SgnLength',{2,8,16,16,16},'SgnType',{0,0,0,0,0},'ModeValue',{-1,-1,-1,-1,-1},'DataType',{0,0,0,0,0},'ByteLayout',{0,0,0,0,0},'Factor',{1,0.05,0.0009765,0.01,3.725e-09},'Offset',{0,0,31.999,0,0.00012206},'SgnComment',{{''},{''},{''},{''},{''}},'SgnUnit',{'','','','',''},'Min',{0,0,0,0,0},'Max',{0,0,0,0,0},'SLDataType',{'SS_DOUBLE','SS_DOUBLE','SS_DOUBLE','SS_DOUBLE','SS_DOUBLE'}),'MsgIdNumFormat',0,'MsgComment',{{''}}),'Version',1.2,'general',struct('isFromLib',0)),'OFF',[]}},'GroupId',{{struct('Group',{{'RTICAN'}},'No',2,'Behavior',{{'NAMECHANGE'}},'BlockType',{{'SINK'}},'NameChangeFlag',0),'OFF',[]}},'SFcnRTICANMessage',{{struct('MsgType','RX','SFcnPortType','Scalar','MsgName','ME_Lane_Additional_Data_3','MsgIdFormat','STD','MsgId',1903,'MsgLength',8,'NumSignals',5,'SampleTime',0.01,'Signal',struct('SgnName',{'Alive_Counter_MELaneAddData','Rh_Neighbor_Pos','Rh_Neighbor_Model_B','Rh_Neighbor_Model_A','Rh_Neighbor_Model_dA'},'SgnStartBit',{0,8,16,32,48},'SgnLength',{2,8,16,16,16},'SgnType',{'standard','standard','standard','standard','standard'},'ModeValue',{-1,-1,-1,-1,-1},'DataType',{['unsigned int'],['unsigned int'],['unsigned int'],['unsigned int'],['unsigned int']},'ByteLayout',{['little endian'],['little endian'],['little endian'],['little endian'],['little endian']},'Factor',{1,0.05,0.0009765,0.01,3.725e-09},'Offset',{0,0,31.999,0,0.00012206},'SLDataType',{'SS_DOUBLE','SS_DOUBLE','SS_DOUBLE','SS_DOUBLE','SS_DOUBLE'}),'StatusSelected','no','TimeSelected','no','DeltaTimeSelected','no','BytePortSelected','no','MessageLengthSelected','no','TriggerPort',struct('Selected','no','TriggerType',0),'UserCoding',struct('Selected','no','InterfaceFile','UserDecodingFile','FcnName','UserDecodeFcn','InportSelected','no','InportWidth',1,'OutportSelected','no','OutportWidth',1),'EnablePortSelected','no','UseRXService','no','BoardType','DS1','BoardNo',1,'ControllerNo',2),'OFF',[]}},'TLCFileName',{{'rtican_rx_message','OFF',[]}})  RTISFcnParameters=struct('SFcnRTICANMessage','struct','TLCFileName','char')  RTIBlockParaDefault=struct('BoardTypeNo',4302,'BoardNo',1,'ChannelNo',1,'Parameters',struct('DataFileSupport',struct('DataFileSelectedMaster',0,'DataFileSelectedLocal',0,'DataFileName','','DataFileDate','','SelectedFile',['<no file selected>']),'Options',struct('StatusSelected',1,'TimeSelected',1,'DeltaTimeSelected',1,'BytePortSelected',0,'MessageLengthSelected',0,'TriggerPort',struct('Selected',0,'TriggerType','rising'),'UserCoding',struct('Selected',0,'InterfaceFile','UserDecodingFile','FcnName','UserDecodeFcn','InportSelected',0,'InportWidth',1,'OutportSelected',0,'OutportWidth',1),'EnablePortSelected',0,'SignalOnPortnameSelected',1,'UseRXService',0),'Message',struct('MsgOnBlocknameSelected',0,'MsgName',['RX Message'],'MsgIdFormat',0,'MsgId',100,'MsgLength',8,'NumSignals',1,'SampleTime',-1,'Signal',struct('SgnName',['RX signal'],'SgnStartBit',0,'SgnLength',8,'SgnType',0,'ModeValue',-1,'DataType',0,'SLDataType','SS_DOUBLE','ByteLayout',0,'Factor',1,'Offset',0,'Min',0,'Max',255,'SgnComment',{{}},'SgnUnit',''),'MsgIdNumFormat',0,'MsgComment',{{''}}),'Version',1.2,'general',struct('isFromLib',1)),'GroupId',struct('Group',{{'RTICAN'}},'No',1,'Behavior',{{'NAMECHANGE'}},'BlockType',{{'SINK'}},'NameChangeFlag',0),'SFcnRTICANMessage',struct('MsgType','RX','MsgName',['RX Message'],'MsgIdFormat','STD','MsgId',100,'MsgLength',8,'NumSignals',1,'SampleTime',-1,'Signal',struct('SgnName',['RX signal'],'SgnStartBit',0,'SgnLength',8,'SgnType','standard','ModeValue',-1,'DataType',['unsigned int'],'ByteLayout',['little endian'],'SLDataType','SS_DOUBLE','Factor',1,'Offset',0),'StatusSelected','yes','TimeSelected','yes','DeltaTimeSelected','yes','BytePortSelected','no','MessageLengthSelected','no','EnablePortSelected','no','UserCoding',struct('Selected','no','InterfaceFile','UserDecodingFile','FcnName','UserDecodeFcn','InportSelected','no','InportWidth',1,'OutportSelected','no','OutportWidth',1),'TriggerPort',struct('Selected','no','TriggerType','rising'),'UseRXService','no','BoardType','DS4302','BoardNo',1,'ControllerNo',1,'SFcnPortType','Scalar'),'TLCFileName','rtican_rx_message')
      settings: AttributesFormatString=Group Id: RTICAN2\n
  ME_Lane_Additional_Data_3_CAN : Outport
  wires:
  Bus Creator/1 -> ME_Lane_Additional_Data_3_CAN/1
  ME_Lane_Additional_Data_3/1 -> Bus Creator/1  "Alive_Counter_MELaneAddData"
  ME_Lane_Additional_Data_3/2 -> Bus Creator/2  "Rh_Neighbor_Pos"
  ME_Lane_Additional_Data_3/3 -> Bus Creator/3  "Rh_Neighbor_Model_B"
  ME_Lane_Additional_Data_3/4 -> Bus Creator/4  "Rh_Neighbor_Model_A"
  ME_Lane_Additional_Data_3/5 -> Bus Creator/5  "Rh_Neighbor_Model_dA"

== system Control_test/InputProcessing/CameraCanProcessing/ME_Left_Lane_A ==
  Bus Creator : BusCreator  Inputs=7
  ME_Left_Lane_A : rtican/RTICAN Receive (RX)   Reserved1=[]  Reserved2=[]  Reserved3=[]  Reserved4=[]  SfcnMessage=[]  Msg_Struct=[]  BoardTypeNo=[]  BoardNo=[]  ChannelNo=[]  Parameters=[]  DialogFcn=[]  UnitName=[]  Revision=[]  UnitValues=[]  DSProperties=struct('RTI',struct('Version',uint32(5),'BlockType',struct('isSLSource',uint8(1),'isSLSink',uint8(1),'isHWSource',uint8(0),'isHWSink',uint8(0),'isSetup',uint8(0),'isInline',uint8(1),'isNonInline',uint8(0),'isInterrupt',uint8(0),'isChannelwise',uint8(0)),'IOBoardType','RTICAN','UnitType','MESSAGE','Identifier','RX','DialogType','MSVC','BlockSet','RTICAN','SlaveProcessor','CAN'))  RTIBlockInterface=struct('OutputPortsWidth',int32([1 1 1 1 1 1 1]),'OutputPortsActive',[1 1 1 1 1 1 1],'OutputPortsName',{{'LaneMarkType_Lh_ME','LaneMarkQuality_Lh_ME','LDW_Warning_Lh_ME','LDW_Availability_Lh_ME','LaneMarkPosition_Lh_ME','LaneMarkModelA_Lh_ME','LaneMarkWidth_Lh_ME'}},'OutputPortsDataType',{{'SS_DOUBLE','SS_DOUBLE','SS_DOUBLE','SS_DOUBLE','SS_DOUBLE','SS_DOUBLE','SS_DOUBLE'}},'OutputPortsLabel',{{'LaneMarkType_Lh_ME','LaneMarkQuality_Lh_ME','LDW_Warning_Lh_ME','LDW_Availability_Lh_ME','LaneMarkPosition_Lh_ME','LaneMarkModelA_Lh_ME','LaneMarkWidth_Lh_ME'}},'OutputPortsLabelMode','ON','InputPortsWidth',int32(0),'InputPortsActive',0,'DialogFcn','rtican_message_interface_gui','BlockDisplay',{{'','center'}},'IconTransparency','on','ParameterTunableNames',{{}},'InitLevel',3,'BlockName',struct('Token',{{'ME_Left_Lane_A'}}),'SampleTime',{{0.01}},'TriggerPort',{{'none'}},'EnablePort',{{'none'}})  RTIBlockParameters=struct('BoardTypeNo',{{1,'OFF',[]}},'BoardNo',{{1,'ON',[1 16]}},'ChannelNo',{{2,'ON',[1 2]}},'Parameters',{{struct('DataFileSupport',struct('DataFileSelectedMaster',1,'DataFileSelectedLocal',0,'DataFileName',['c:\users\mpc\dropbox\cpg_test_2014\t4_rfs_demo\hyundai car setup\rt2000_can_mod.dbc|c:\users\mpc\dropbox\cpg_test_2014\t4_rfs_demo\hyundai car setup\mobileye spec new\mobileye_mando_camera_ucb_v2.dbc|'],'DataFileDate',{{{['13-Nov-2012 16:29:35']},{['18-Sep-2013 10:55:24']}}},'SelectedFile',['<no file selected>'],'InterfaceFcn','rtican_dbc_file_parser'),'Options',struct('StatusSelected',0,'TimeSelected',0,'DeltaTimeSelected',0,'BytePortSelected',0,'MessageLengthSelected',0,'TriggerPort',struct('Selected',0,'TriggerType',0),'UserCoding',struct('Selected',0,'InterfaceFile','UserDecodingFile','FcnName','UserDecodeFcn','InportSelected',0,'InportWidth',1,'OutportSelected',0,'OutportWidth',1),'EnablePortSelected',0,'SignalOnPortnameSelected',1,'UseRXService',0),'Message',struct('MsgOnBlocknameSelected',1,'MsgName','ME_Left_Lane_A','MsgIdFormat',0,'MsgId',1894,'MsgLength',8,'NumSignals',7,'SampleTime',0.01,'Signal',struct('SgnName',{'LaneMarkType_Lh_ME','LaneMarkQuality_Lh_ME','LDW_Warning_Lh_ME','LDW_Availability_Lh_ME','LaneMarkPosition_Lh_ME','LaneMarkModelA_Lh_ME','LaneMarkWidth_Lh_ME'},'SgnStartBit',{0,4,6,7,8,24,56},'SgnLength',{4,2,1,1,16,32,8},'SgnType',{0,0,0,0,0,0,0},'ModeValue',{-1,-1,-1,-1,-1,-1,-1},'DataType',{0,0,0,0,1,0,0},'ByteLayout',{0,0,0,0,0,0,0},'Factor',{1,1,1,1,0.00390625,2.3283064e-10,0.005},'Offset',{0,0,0,0,0,-0.5,0},'SgnComment',{{''},{''},{''},{''},{''},{''},{''}},'SgnUnit',{'','','','','','1/Meters',''},'Min',{0,0,0,0,0,0,0},'Max',{0,0,0,0,0,0,0},'SLDataType',{'SS_DOUBLE','SS_DOUBLE','SS_DOUBLE','SS_DOUBLE','SS_DOUBLE','SS_DOUBLE','SS_DOUBLE'}),'MsgIdNumFormat',1,'MsgComment',{{''}}),'Version',1.2,'general',struct('isFromLib',0)),'OFF',[]}},'GroupId',{{struct('Group',{{'RTICAN'}},'No',2,'Behavior',{{'NAMECHANGE'}},'BlockType',{{'SINK'}},'NameChangeFlag',0),'OFF',[]}},'SFcnRTICANMessage',{{struct('MsgType','RX','SFcnPortType','Scalar','MsgName','ME_Left_Lane_A','MsgIdFormat','STD','MsgId',1894,'MsgLength',8,'NumSignals',7,'SampleTime',0.01,'Signal',struct('SgnName',{'LaneMarkType_Lh_ME','LaneMarkQuality_Lh_ME','LDW_Warning_Lh_ME','LDW_Availability_Lh_ME','LaneMarkPosition_Lh_ME','LaneMarkModelA_Lh_ME','LaneMarkWidth_Lh_ME'},'SgnStartBit',{0,4,6,7,8,24,56},'SgnLength',{4,2,1,1,16,32,8},'SgnType',{'standard','standard','standard','standard','standard','standard','standard'},'ModeValue',{-1,-1,-1,-1,-1,-1,-1},'DataType',{['unsigned int'],['unsigned int'],['unsigned int'],['unsigned int'],['signed int'],['unsigned int'],['unsigned int']},'ByteLayout',{['little endian'],['little endian'],['little endian'],['little endian'],['little endian'],['little endian'],['little endian']},'Factor',{1,1,1,1,0.00390625,2.3283064e-10,0.005},'Offset',{0,0,0,0,0,-0.5,0},'SLDataType',{'SS_DOUBLE','SS_DOUBLE','SS_DOUBLE','SS_DOUBLE','SS_DOUBLE','SS_DOUBLE','SS_DOUBLE'}),'StatusSelected','no','TimeSelected','no','DeltaTimeSelected','no','BytePortSelected','no','MessageLengthSelected','no','TriggerPort',struct('Selected','no','TriggerType',0),'UserCoding',struct('Selected','no','InterfaceFile','UserDecodingFile','FcnName','UserDecodeFcn','InportSelected','no','InportWidth',1,'OutportSelected','no','OutportWidth',1),'EnablePortSelected','no','UseRXService','no','BoardType','DS1','BoardNo',1,'ControllerNo',2),'OFF',[]}},'TLCFileName',{{'rtican_rx_message','OFF',[]}})  RTISFcnParameters=struct('SFcnRTICANMessage','struct','TLCFileName','char')  RTIBlockParaDefault=struct('BoardTypeNo',4302,'BoardNo',1,'ChannelNo',1,'Parameters',struct('DataFileSupport',struct('DataFileSelectedMaster',0,'DataFileSelectedLocal',0,'DataFileName','','DataFileDate','','SelectedFile',['<no file selected>']),'Options',struct('StatusSelected',1,'TimeSelected',1,'DeltaTimeSelected',1,'BytePortSelected',0,'MessageLengthSelected',0,'TriggerPort',struct('Selected',0,'TriggerType','rising'),'UserCoding',struct('Selected',0,'InterfaceFile','UserDecodingFile','FcnName','UserDecodeFcn','InportSelected',0,'InportWidth',1,'OutportSelected',0,'OutportWidth',1),'EnablePortSelected',0,'SignalOnPortnameSelected',1,'UseRXService',0),'Message',struct('MsgOnBlocknameSelected',0,'MsgName',['RX Message'],'MsgIdFormat',0,'MsgId',100,'MsgLength',8,'NumSignals',1,'SampleTime',-1,'Signal',struct('SgnName',['RX signal'],'SgnStartBit',0,'SgnLength',8,'SgnType',0,'ModeValue',-1,'DataType',0,'SLDataType','SS_DOUBLE','ByteLayout',0,'Factor',1,'Offset',0,'Min',0,'Max',255,'SgnComment',{{}},'SgnUnit',''),'MsgIdNumFormat',0,'MsgComment',{{''}}),'Version',1.2,'general',struct('isFromLib',1)),'GroupId',struct('Group',{{'RTICAN'}},'No',1,'Behavior',{{'NAMECHANGE'}},'BlockType',{{'SINK'}},'NameChangeFlag',0),'SFcnRTICANMessage',struct('MsgType','RX','MsgName',['RX Message'],'MsgIdFormat','STD','MsgId',100,'MsgLength',8,'NumSignals',1,'SampleTime',-1,'Signal',struct('SgnName',['RX signal'],'SgnStartBit',0,'SgnLength',8,'SgnType','standard','ModeValue',-1,'DataType',['unsigned int'],'ByteLayout',['little endian'],'SLDataType','SS_DOUBLE','Factor',1,'Offset',0),'StatusSelected','yes','TimeSelected','yes','DeltaTimeSelected','yes','BytePortSelected','no','MessageLengthSelected','no','EnablePortSelected','no','UserCoding',struct('Selected','no','InterfaceFile','UserDecodingFile','FcnName','UserDecodeFcn','InportSelected','no','InportWidth',1,'OutportSelected','no','OutportWidth',1),'TriggerPort',struct('Selected','no','TriggerType','rising'),'UseRXService','no','BoardType','DS4302','BoardNo',1,'ControllerNo',1,'SFcnPortType','Scalar'),'TLCFileName','rtican_rx_message')
      settings: AttributesFormatString=Group Id: RTICAN2\n
  ME_Left_Lane_A_CAN : Outport
  wires:
  Bus Creator/1 -> ME_Left_Lane_A_CAN/1
  ME_Left_Lane_A/1 -> Bus Creator/1  "LaneMarkType_Lh_ME"
  ME_Left_Lane_A/2 -> Bus Creator/2  "LaneMarkQuality_Lh_ME"
  ME_Left_Lane_A/3 -> Bus Creator/3  "LDW_Warning_Lh_ME"
  ME_Left_Lane_A/4 -> Bus Creator/4  "LDW_Availability_Lh_ME"
  ME_Left_Lane_A/5 -> Bus Creator/5  "LaneMarkPosition_Lh_ME"
  ME_Left_Lane_A/6 -> Bus Creator/6  "LaneMarkModelA_Lh_ME"
  ME_Left_Lane_A/7 -> Bus Creator/7  "LaneMarkWidth_Lh_ME"
